simulink model "ball_and_beam_fuzzy"  (R2024b)
settings: Solver=ode45  StartTime=0  StopTime=50  MaxStep=0.4  RelTol=1e-3  AbsTol=1e-6
PreLoadFcn:
  | tank=readfis('tank');
values from neighbouring files (symbols this model uses):
  g = 9.8    [Beam_Parameters.m]    (also in animballandbeam.m = 0.05)
  J = (1/12) * mb * L^2    (= 0.16875)    [Beam_Parameters.m]
  L = 3    [Beam_Parameters.m]
  m = 0.11    [Beam_Parameters.m]
  R = 0.15    [Beam_Parameters.m]
libraries: fuzblock x1
CloseFcn:
  | AnimFigH = findobj(0,'Name', 'Tank Demo'); close(AnimFigH)
settings Model: PacingRate=4  Creator=pascal  LastModifiedBy=TRANKHOINGUYEN
settings SolverCC: AutoScaleAbsTol=off  ZeroCrossAlgorithm=Adaptive  AlgebraicLoopSolver=TrustRegion
settings DataIOCC: SaveFormat=Array  SignalLoggingSaveFormat=ModelDataLogs  SaveOutput=off  SaveTime=off  ReturnWorkspaceOutputs=off
settings OptimizationCC: BlockReduction=off  BooleanDataType=off  ExpressionDepthLimit=2147483647  InitFltsAndDblsToZero=on  LifeSpan=inf
settings DebuggingCC: SaveWithParameterizedLinksMsg=none  UnderspecifiedInitializationDetection=Classic  MergeDetectMultiDrivingBlocksExec=none  SignalResolutionControl=TryResolveAllWithWarning  IgnoredZcDiagnostic=none  MultiTaskDSMMsg=warning  MultiTaskCondExecSysMsg=none  FcnCallInpInsideContextMsg=warning  UnconnectedInputMsg=warning  UnconnectedOutputMsg=warning  UnconnectedLineMsg=warning  StateNameClashWarn=warning  SFUnexpectedBacktrackingDiag=warning  SFNoUnconditionalDefaultTransitionDiag=warning  SFExecutionAtInitializationDiag=none  ArithmeticOperatorsInVariantConditions=warning
settings HardwareCC: ProdBitPerPointer=32  ProdBitPerSizeT=32  ProdBitPerPtrDiffT=32  ProdLargestAtomicFloat=None  ProdIntDivRoundTo=Undefined  ProdEndianess=Unspecified  ProdWordSize=32  ProdHWDeviceType=32-bit Generic  TargetBitPerPointer=64  TargetBitPerSizeT=64  TargetBitPerPtrDiffT=64  TargetLongLongMode=on  TargetIntDivRoundTo=Zero  TargetEndianess=LittleEndian  TargetWordSize=64  TargetHWDeviceType=MATLAB Host  ProdEqTarget=off
settings ModelReferenceCC: EnableRefExpFcnMdlSchedulingChecks=on  PropagateSignalLabelsOutOfModel=off
settings SFSimCC: SimUseLocalCustomCode=off  CustomCodeUndefinedFunction=UseInterfaceOnly
settings RTWCC: GenerateMakefile=off  TemplateMakefile=grt_unix.tmf  RTWUseLocalCustomCode=off  GPUComputeCapability=3.5
settings CodeAppCC: StateflowObjectComments=on
settings GRTTargetCC: TargetFcnLib=ansi_tfl_tmw.mat  TargetLangStandard=C89/C90 (ANSI)  CombineOutputUpdateFcns=off  GRTInterface=on
settings ConfigComp: CovMetricSettings=dw  CovSaveCumulativeToWorkspaceVar=on  CovSaveSingleToWorkspaceVar=on  CovExternalEMLEnable=off

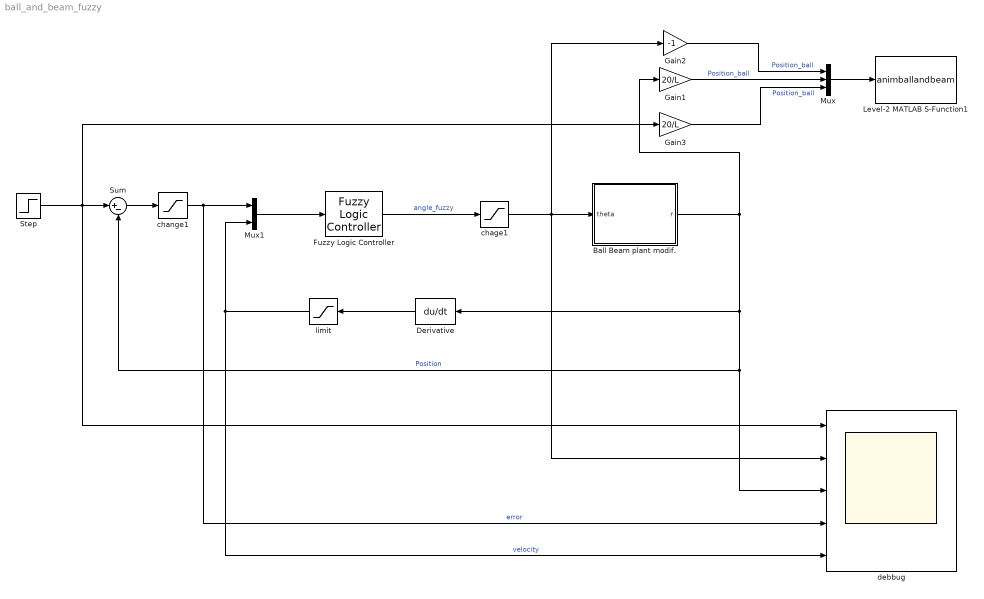
== system ball_and_beam_fuzzy ==
  Ball Beam plant modif. : Subsystem
  Derivative : Derivative  CoefficientInTFapproximation=100000000
  Fuzzy Logic Controller : fuzblock/Fuzzy Logic  Controller  FIS='ball_and_beam_Fuzzy.fis'  OutputSampleNumber=101  DataType=double  FuzzifiedInputs=off  RuleFiringStrengths=off  RuleOutputs=off  AggregatedOutputs=off  SimulateUsing=Interpreted execution  OutOfRangeInputValueMessage=warning  NoRuleFiredMessage=warning  EmptyOutputFuzzySetMessage=warning
  Gain1 : Gain  Gain=20/L
  Gain2 : Gain  Gain=-1
  Gain3 : Gain  Gain=20/L
  Level-2 MATLAB S-Function1 : M-S-Function  FunctionName=animballandbeam  Parameters=1
  Mux : Mux  Inputs=3
  Mux1 : Mux  Inputs=2
  Step : Step  SampleTime=0
  Sum : Sum  Inputs=|+-
  chage1 : Saturate  UpperLimit=0.2617  LowerLimit=-0.2617
  change1 : Saturate  UpperLimit=1  LowerLimit=-1
  debbug : Scope  NumInputPorts=5
  limit : Saturate  UpperLimit=0.1  LowerLimit=-0.1
  wires:
  Derivative/1 -> limit/1
  Mux1/1 -> Fuzzy Logic Controller/1
  limit/1 -> debbug/5, Mux1/2  "velocity"
  Fuzzy Logic Controller/1 -> chage1/1  "angle_fuzzy"
  change1/1 -> debbug/4, Mux1/1  "error"
  Sum/1 -> change1/1
  Ball Beam plant modif./1(r) -> Gain1/1, debbug/3, Sum/2, Derivative/1  "Position"
  Step/1 -> debbug/1, Gain3/1, Sum/1
  Mux/1 -> Level-2 MATLAB S-Function1/1
  Gain1/1 -> Mux/2  "Position_ball"
  Gain3/1 -> Mux/3  "Position_ball"
  chage1/1 -> debbug/2, Gain2/1, Ball Beam plant modif./1(theta)
  Gain2/1 -> Mux/1  "Position_ball"

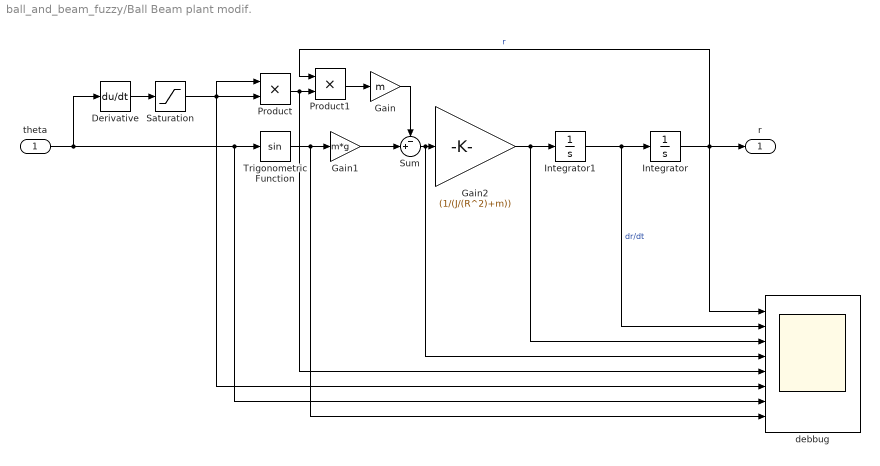
== system ball_and_beam_fuzzy/Ball Beam plant modif. ==
  theta : Inport
  Derivative : Derivative  CoefficientInTFapproximation=1000
  Gain : Gain  Gain=m
  Gain1 : Gain  Gain=m*g
  Gain2 : Gain  Gain=(1/(J/(R^2)+m))
  Integrator : Integrator
  Integrator1 : Integrator
  Product : Product
  Product1 : Product
  Saturation : Saturate  LinearizeAsGain=off  ZeroCross=off
  Sum : Sum  Inputs=-+|
  Trigonometric Function : Trigonometry
  debbug : Scope  NumInputPorts=8
  r : Outport
  wires:
  Derivative/1 -> Saturation/1
  Integrator1/1 -> debbug/2, Integrator/1  "dr/dt"
  Integrator/1 -> debbug/1, Product1/1, r/1  "r"
  theta/1 -> debbug/7, Trigonometric Function/1, Derivative/1
  Gain2/1 -> debbug/3, Integrator1/1
  Product/1 -> debbug/5, Product1/2
  Product1/1 -> Gain/1
  Sum/1 -> debbug/4, Gain2/1
  Trigonometric Function/1 -> debbug/8, Gain1/1
  Gain1/1 -> Sum/2
  Gain/1 -> Sum/1
  Saturation/1 -> Product/1, debbug/6, Product/2
